simulink model "FlightTable_HWInterface_CC"  (R2019b)
settings: Solver=ode3  StartTime=0.0  StopTime=inf  FixedStep=FT_HWI_CC_Data.SampTime  RelTol=1e-3  EnableMultiTasking=on
undefined symbols (not defined in the file or in its folder): FT_HWI_CC_Data
libraries: lib_Gimbal_Ctrl x3, simulink x2, lib_Gimbal x1
settings Model: SimulationMode=external  Creator=sasson  LastModifiedBy=guy-m
settings DataIOCC: MaxDataPoints=100000  SaveFormat=Array  SaveState=on  SignalLogging=off  VisualizeSimOutput=off  ReturnWorkspaceOutputs=off
settings DebuggingCC: SFUnexpectedBacktrackingDiag=warning  SFNoUnconditionalDefaultTransitionDiag=warning  SFExecutionAtInitializationDiag=none  ArithmeticOperatorsInVariantConditions=warning
settings HardwareCC: TargetBitPerLong=64  TargetBitPerPointer=64  TargetIntDivRoundTo=Zero  TargetEndianess=LittleEndian  TargetWordSize=64  TargetHWDeviceType=Intel->x86-64
settings ModelReferenceCC: PropagateSignalLabelsOutOfModel=off
settings SFSimCC: SimUseLocalCustomCode=off  CustomCodeUndefinedFunction=UseInterfaceOnly
settings RTWCC: Description=Simulink Desktop Real-Time  SystemTargetFile=sldrt.tlc  TemplateMakefile=sldrt.tmf  RTWUseLocalCustomCode=off  RTWCompilerOptimization=on
settings CodeAppCC: MaxIdLength=95  StateflowObjectComments=on
settings SimulinkDesktopRealTimeCC: TargetPreCompLibLocation=C:\Program Files\MATLAB\R2019b\toolbox\sldrt\lib\win64  TargetLangStandard=C89/C90 (ANSI)  SupportVariableSizeSignals=off  PreserveStateflowLocalDataDimensions=off
settings ConfigComp: CovMetricSettings=dw  CovHtmlReporting=on  CovSaveCumulativeToWorkspaceVar=on  CovSaveSingleToWorkspaceVar=on  CovExternalEMLEnable=off

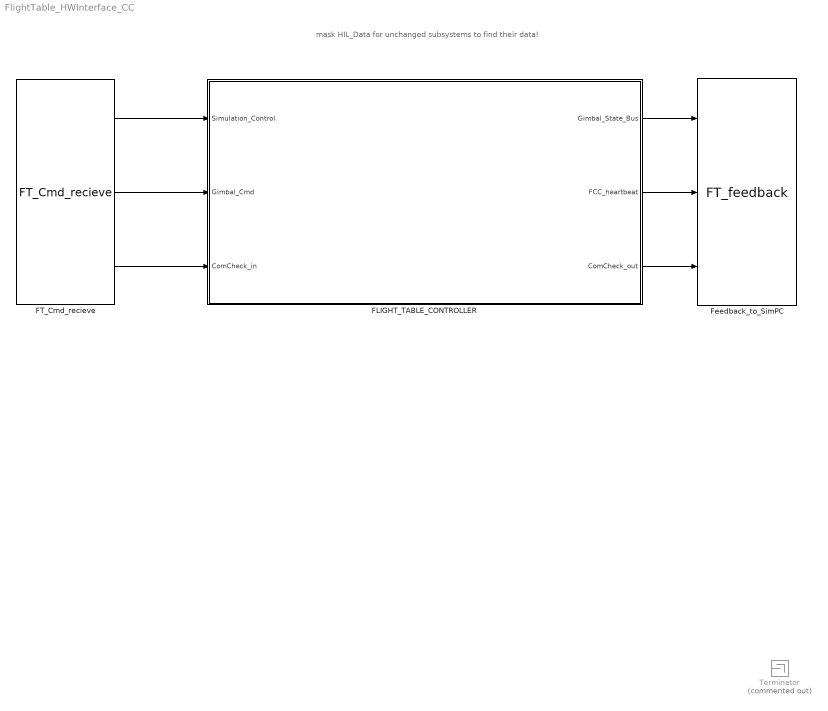
== system FlightTable_HWInterface_CC ==
  note: mask HIL_Data for unchanged subsystems to find their data!
  FLIGHT_TABLE_CONTROLLER : Subsystem  mask{HIL_Data=FT_HWI_CC_Data.HIL_Data}
      mask prompts: HIL_Data "Mimic HIL_Data"
  FT_Cmd_recieve : lib_Gimbal_Ctrl/FT_Cmd_recieve  SystemSampleTime=-1  Latency=0  AutoFrameSizeCalculation=off
  Feedback_to_SimPC : lib_Gimbal_Ctrl/FT_feedback  SystemSampleTime=-1  Latency=0  AutoFrameSizeCalculation=off
  Terminator : Terminator  Commented=on
  wires:
  ? -> Terminator/1
  FT_Cmd_recieve/2 -> FLIGHT_TABLE_CONTROLLER/2(Gimbal_Cmd)
  FT_Cmd_recieve/1 -> FLIGHT_TABLE_CONTROLLER/1(Simulation_Control)
  FLIGHT_TABLE_CONTROLLER/1(Gimbal_State_Bus) -> Feedback_to_SimPC/1
  FT_Cmd_recieve/3 -> FLIGHT_TABLE_CONTROLLER/3(ComCheck_in)
  FLIGHT_TABLE_CONTROLLER/2(FCC_heartbeat) -> Feedback_to_SimPC/2
  FLIGHT_TABLE_CONTROLLER/3(ComCheck_out) -> Feedback_to_SimPC/3

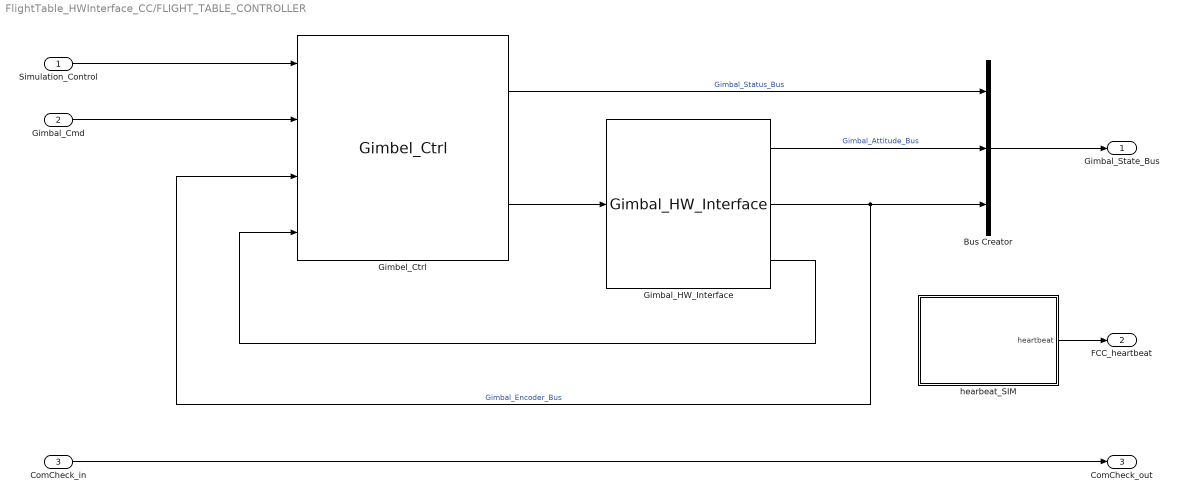
== system FlightTable_HWInterface_CC/FLIGHT_TABLE_CONTROLLER ==
  Simulation_Control : Inport  OutDataTypeStr=Bus: Simulation_Ctrl_Bus
  Gimbal_Cmd : Inport  Port=2  OutDataTypeStr=Bus: Gimbal_Cmd_Bus
  ComCheck_in : Inport  Port=3
  Bus Creator : BusCreator  Inputs=3  OutDataTypeStr=Bus: Gimbal_State_Bus
  Gimbal_HW_Interface : lib_Gimbal/Gimbal_HW_Interface  HW=HIL_Data.Gimbal.HW
      link override Encoder Input3: SampleTime=HW.SampTime  MaxMissedTicks=HW.MaxMissTick  ShowMissedTicks=off  YieldWhenWaiting=off  DrvName=National_Instruments/PCIe-6353  DrvAddress=4294967295  DrvOptions=[0 15 0 2 2 2 2]  Channels=[1:3]  QuadMode=3  IndexPulse=1  InputFilter=Inf  DataType=1
  Gimbel_Ctrl : lib_Gimbal_Ctrl/Gimbel_Ctrl  Gimbal_Ctrl=HIL_Data.Gimbal_Ctrl  SampTime=HIL_Data.Gimbal_Ctrl.SampTime
  hearbeat_SIM : Subsystem
  Gimbal_State_Bus : Outport  OutDataTypeStr=Bus: Gimbal_State_Bus
  FCC_heartbeat : Outport  Port=2
  ComCheck_out : Outport  Port=3
  wires:
  Gimbel_Ctrl/2 -> Gimbal_HW_Interface/1
  Gimbel_Ctrl/1 -> Bus Creator/1  "Gimbal_Status_Bus"
  Gimbal_HW_Interface/1 -> Bus Creator/2  "Gimbal_Attitude_Bus"
  Gimbal_HW_Interface/2 -> Gimbel_Ctrl/3, Bus Creator/3  "Gimbal_Encoder_Bus"
  Gimbal_HW_Interface/3 -> Gimbel_Ctrl/4
  Gimbal_Cmd/1 -> Gimbel_Ctrl/2
  Simulation_Control/1 -> Gimbel_Ctrl/1
  Bus Creator/1 -> Gimbal_State_Bus/1
  hearbeat_SIM/1(heartbeat) -> FCC_heartbeat/1
  ComCheck_in/1 -> ComCheck_out/1

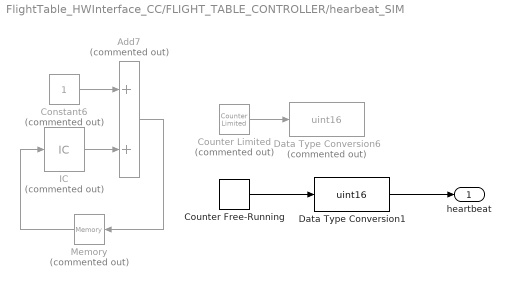
== system FlightTable_HWInterface_CC/FLIGHT_TABLE_CONTROLLER/hearbeat_SIM ==
  Add7 : Sum  Commented=on
  Constant6 : Constant  Commented=on
  Counter Free-Running : simulink/Sources/Counter Free-Running  NumBits=FT_HWI_CC_Data.heartbeat.range  tsamp=FT_HWI_CC_Data.SampTime
  Counter Limited : simulink/Sources/Counter Limited  Commented=on  uplimit=50000  tsamp=-1
  Data Type Conversion1 : DataTypeConversion  OutDataTypeStr=uint16
  Data Type Conversion6 : DataTypeConversion  Commented=on  OutDataTypeStr=uint16
  IC : InitialCondition  Commented=on  Value=0
  Memory : Memory  Commented=on  InheritSampleTime=on
  heartbeat : Outport
  wires:
  Add7/1 -> Memory/1
  IC/1 -> Add7/2
  Memory/1 -> IC/1
  Constant6/1 -> Add7/1
  Counter Limited/1 -> Data Type Conversion6/1
  Counter Free-Running/1 -> Data Type Conversion1/1
  Data Type Conversion1/1 -> heartbeat/1
